simulink model "stellaris_lp_blink_bluetooth"  (R2017b)
settings: Solver=FixedStepDiscrete  StartTime=0.0  StopTime=10.0  FixedStep=0.0001  RelTol=1e-3
libraries: stellaris_lp_lib x8, etargetslib x1, xpcutilitieslib x1
settings Model: ExtModeTrigDuration=2  Creator=peselnikmg  LastModifiedBy=Mitchell Cassaday
settings DataIOCC: LimitDataPoints=on  SaveFormat=Array  SignalLoggingSaveFormat=ModelDataLogs  ReturnWorkspaceOutputs=on
settings OptimizationCC: UseDivisionForNetSlopeComputation=on  UseFloatMulNetSlope=on  UseSpecifiedMinMax=on  PassReuseOutputArgsAs=Individual arguments  ExpressionDepthLimit=2147483647  ZeroExternalMemoryAtStartup=off  ZeroInternalMemoryAtStartup=off  NoFixptDivByZeroProtection=on  EfficientFloat2IntCast=on  LifeSpan=inf  MaxStackSize=64  OptimizeBlockOrder=speed
settings DebuggingCC: ReadBeforeWriteMsg=DisableAll  WriteAfterWriteMsg=DisableAll  WriteAfterReadMsg=DisableAll  MultiTaskDSMMsg=none  IntegerOverflowMsg=error  ParameterTunabilityLossMsg=error  AssertControl=DisableAll  StateNameClashWarn=warning  NonBusSignalsTreatedAsBus=error  SFInvalidInputDataAccessInChartInitDiag=error  SFTransitionOutsideNaturalParentDiag=error  SFUnreachableExecutionPathDiag=error  SFUndirectedBroadcastEventsDiag=error  SFExecutionAtInitializationDiag=none  IntegerSaturationMsg=error
settings HardwareCC: ProdBitPerPointer=32  ProdBitPerSizeT=32  ProdBitPerPtrDiffT=32  ProdLargestAtomicInteger=Long  ProdLargestAtomicFloat=Double  ProdWordSize=32  ProdHWDeviceType=ARM Compatible->ARM Cortex
settings ModelReferenceCC: UpdateModelReferenceTargets=IfOutOfDate  PropagateSignalLabelsOutOfModel=off
settings SFSimCC: SFSimEcho=off  MATLABDynamicMemAlloc=off
settings RTWCC: SystemTargetFile=ert.tlc  HardwareBoard=Tiva TM4C123G Launchpad  TLCOptions=-aInlineSetEventsForThisBaseRateFcn=TLC_FALSE -aSuppressMultiTaskScheduler=TLC_FALSE -aRateBasedStepFcn=1  TemplateMakefile=ert_default_tmf  GenerateReport=on  RTWVerbose=off  Toolchain=Texas Instruments Code Composer Studio (Tiva)  BuildConfiguration=Faster Runs  IncludeHyperlinkInReport=on  LaunchReport=on  GenerateTraceInfo=on  GenerateTraceReport=on  GenerateTraceReportSl=on  GenerateTraceReportSf=on  GenerateTraceReportEml=on
settings CodeAppCC: ForceParamTrailComments=on  IgnoreCustomStorageClasses=off  OperatorAnnotations=on  SimulinkDataObjDesc=on  SFDataObjDesc=on  MATLABFcnDesc=on  CustomSymbolStrType=$N$R$M  InsertBlockDesc=on  StateflowObjectComments=on  MATLABSourceComments=on  EnableCustomComments=on  ReqsInCode=on
settings ERTTargetCC: UtilityFuncGeneration=Shared location  CombineSignalStateStructs=on  SuppressErrorStatus=on  SupportNonFinite=off  ParenthesesLevel=Maximum  CastingMode=Standards  EnableSignedLeftShifts=off  EnableSignedRightShifts=off
settings ConfigComp: CovMetricSettings=dw  CovHtmlReporting=on  CovSaveCumulativeToWorkspaceVar=on  CovSaveSingleToWorkspaceVar=on  CovExternalEMLEnable=off

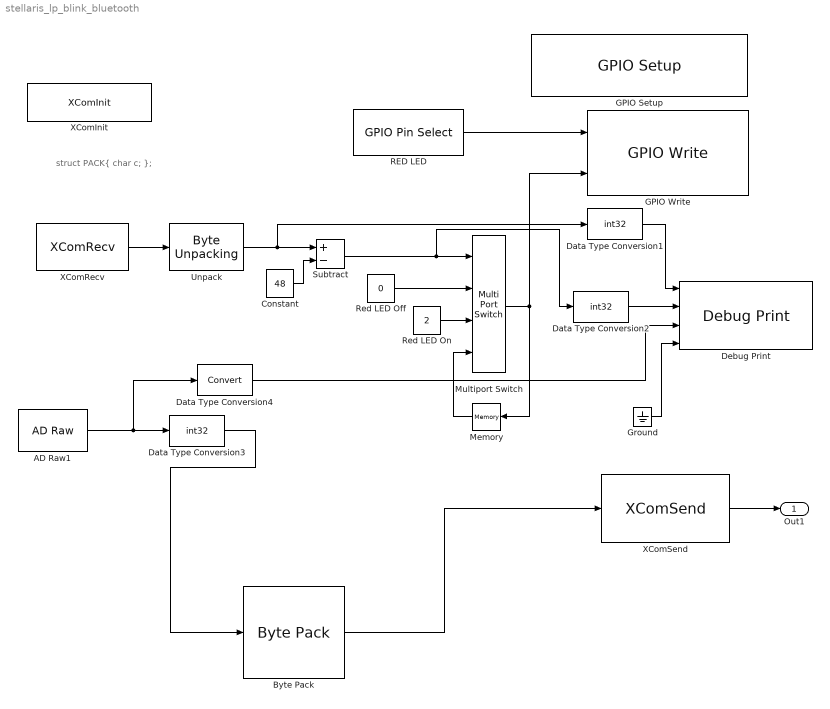
== system stellaris_lp_blink_bluetooth ==
  note: struct  PACK{
      | 		char c;
      | };
  AD Raw1 : stellaris_lp_lib/ADC/AD Raw  ch="2   PE2"  sample_time=.02
      settings: SourceProductName=Run on Stellaris LaunchPad
  Byte Pack : etargetslib/Byte Pack  datatypes={'int32'}  byteAlign=1
  Constant : Constant  Value=48  OutDataTypeStr=uint8
  Data Type Conversion1 : DataTypeConversion  OutDataTypeStr=int32
  Data Type Conversion2 : DataTypeConversion  OutDataTypeStr=int32
  Data Type Conversion3 : DataTypeConversion  OutDataTypeStr=int32
  Data Type Conversion4 : DataTypeConversion
  Debug Print : stellaris_lp_lib/Debug/Debug Print  fmt="'Convert %d    Distance  %d    min  %d    max  %d'"  sample_time=-1
      settings: SourceProductName=Run on Stellaris LaunchPad
  GPIO Setup : stellaris_lp_lib/GPIO/GPIO Setup  GPIO_PORTX_BASE=GPIO_PORTF_BASE  PinsOutput_0=Input  PinsOutput_1=Output  PinsOutput_2=Output  PinsOutput_3=Output  PinsOutput_4=Input  PinsOutput_5=Input  PinsOutput_6=Input  PinsOutput_7=Input
      settings: SourceProductName=Run on Stellaris LaunchPad
  GPIO Write : stellaris_lp_lib/GPIO/GPIO Write  GPIO_PORTX_BASE=GPIO_PORTF_BASE  SampleTime=-1
      settings: SourceProductName=Run on Stellaris LaunchPad
  Ground : Ground
  Memory : Memory
  Multiport Switch : MultiPortSwitch  DataPortOrder=Zero-based contiguous  DiagnosticForDefault=None
  RED LED : stellaris_lp_lib/GPIO/GPIO Pin Select  GPIO_PIN_X=GPIO_PIN_1
      settings: SourceProductName=Run on Stellaris LaunchPad
  Red LED Off : Constant  Value=0  OutDataTypeStr=uint8
  Red LED On : Constant  Value=2  OutDataTypeStr=uint8
  Subtract : Sum  Inputs=+-
  Unpack : xpcutilitieslib/Byte Unpacking   MaskUnpackedDataTypes={'uint8'}  MaskUnpackedDataSizes={1}  MaskAlignment=1
      settings: SourceProductName=Simulink Real-Time  SourceProductBaseCode=XP
  XComInit : stellaris_lp_lib/Communication/XComInit  baud=9600
      settings: SourceProductName=Run on Stellaris LaunchPad
  XComRecv : stellaris_lp_lib/Communication/XComRecv  pack_size=1  sample_time=0.2
      settings: SourceProductName=Run on Stellaris LaunchPad
  XComSend : stellaris_lp_lib/Communication/XComSend  pack_size=4  sample_time=.04
      settings: SourceProductName=Run on Stellaris LaunchPad
  Out1 : Outport
  wires:
  RED LED/1 -> GPIO Write/1
  XComRecv/1 -> Unpack/1
  Multiport Switch/1 -> Memory/1, GPIO Write/2
  Unpack/1 -> Data Type Conversion1/1, Subtract/1
  Constant/1 -> Subtract/2
  Subtract/1 -> Data Type Conversion2/1, Multiport Switch/1
  Red LED Off/1 -> Multiport Switch/2
  Red LED On/1 -> Multiport Switch/3
  Memory/1 -> Multiport Switch/4
  Data Type Conversion1/1 -> Debug Print/1
  Data Type Conversion2/1 -> Debug Print/2
  Data Type Conversion3/1 -> Byte Pack/1
  AD Raw1/1 -> Data Type Conversion4/1, Data Type Conversion3/1
  Ground/1 -> Debug Print/4
  Byte Pack/1 -> XComSend/1
  XComSend/1 -> Out1/1
  Data Type Conversion4/1 -> Debug Print/3
